simulink model "matlab_physics_demo_model"  (R2022b)
settings: Solver=ode4  StartTime=0.0  StopTime=inf  FixedStep=0.003  RelTol=1e-3
values from neighbouring files (symbols this model uses):
  A1 = 0    [load_quadrotor_simulink_combined_model.m]    (also in load_quadrotor_simulink_physics_model.m; load_quadtiltrotor_simulink_physics_model.m = 0.007)
  Apolar = 0    [load_quadrotor_simulink_combined_model.m]    (also in load_quadrotor_simulink_physics_model.m; load_quadtiltrotor_simulink_physics_model.m = 0.057)
  CD0 = 0    [load_quadrotor_simulink_combined_model.m]    (also in load_quadrotor_simulink_physics_model.m; load_quadtiltrotor_simulink_physics_model.m = 0.022)
  chord = 1    [load_quadrotor_simulink_combined_model.m]    (also in load_quadrotor_simulink_physics_model.m; load_quadtiltrotor_simulink_physics_model.m = 0.351342)
  CL0 = 0    [load_quadrotor_simulink_combined_model.m]    (also in load_quadrotor_simulink_physics_model.m; load_quadtiltrotor_simulink_physics_model.m = 0.38)
  CLa = 0    [load_quadrotor_simulink_combined_model.m]    (also in load_quadrotor_simulink_physics_model.m; load_quadtiltrotor_simulink_physics_model.m = 18.5)
  CLa_dot = 0    [load_quadrotor_simulink_combined_model.m]    (also in load_quadrotor_simulink_physics_model.m; load_quadtiltrotor_simulink_physics_model.m = 2.64)
  Clb = 0    [load_quadrotor_simulink_combined_model.m]    (also in load_quadrotor_simulink_physics_model.m; load_quadtiltrotor_simulink_physics_model.m)
  ClDa = 0    [load_quadrotor_simulink_combined_model.m]    (also in load_quadrotor_simulink_physics_model.m; load_quadtiltrotor_simulink_physics_model.m = 0.1695)
  CLDe = 0    [load_quadrotor_simulink_combined_model.m]    (also in load_quadrotor_simulink_physics_model.m; load_quadtiltrotor_simulink_physics_model.m)
  CLDf = 0    [load_quadrotor_simulink_combined_model.m]    (also in load_quadrotor_simulink_physics_model.m; load_quadtiltrotor_simulink_physics_model.m = 0.4)
  ClDr = 0    [load_quadrotor_simulink_combined_model.m]    (also in load_quadrotor_simulink_physics_model.m; load_quadtiltrotor_simulink_physics_model.m)
  Clp = 0    [load_quadrotor_simulink_combined_model.m]    (also in load_quadrotor_simulink_physics_model.m; load_quadtiltrotor_simulink_physics_model.m)
  CLq = 0    [load_quadrotor_simulink_combined_model.m]    (also in load_quadrotor_simulink_physics_model.m; load_quadtiltrotor_simulink_physics_model.m = 7.4)
  Clr = 0    [load_quadrotor_simulink_combined_model.m]    (also in load_quadrotor_simulink_physics_model.m; load_quadtiltrotor_simulink_physics_model.m)
  Cm0 = 0    [load_quadrotor_simulink_combined_model.m]    (also in load_quadrotor_simulink_physics_model.m; load_quadtiltrotor_simulink_physics_model.m)
  Cma = 0    [load_quadrotor_simulink_combined_model.m]    (also in load_quadrotor_simulink_physics_model.m; load_quadtiltrotor_simulink_physics_model.m)
  CmDe = 0    [load_quadrotor_simulink_combined_model.m]    (also in load_quadrotor_simulink_physics_model.m; load_quadtiltrotor_simulink_physics_model.m = -3.2)
  CmDf = 0    [load_quadrotor_simulink_combined_model.m]    (also in load_quadrotor_simulink_physics_model.m; load_quadtiltrotor_simulink_physics_model.m)
  Cmq = 0    [load_quadrotor_simulink_combined_model.m]    (also in load_quadrotor_simulink_physics_model.m; load_quadtiltrotor_simulink_physics_model.m)
  Cnb = 0    [load_quadrotor_simulink_combined_model.m]    (also in load_quadrotor_simulink_physics_model.m; load_quadtiltrotor_simulink_physics_model.m)
  CnDa = 0    [load_quadrotor_simulink_combined_model.m]    (also in load_quadrotor_simulink_physics_model.m; load_quadtiltrotor_simulink_physics_model.m = -0.023)
  CnDr = 0    [load_quadrotor_simulink_combined_model.m]    (also in load_quadrotor_simulink_physics_model.m; load_quadtiltrotor_simulink_physics_model.m)
  Cnp = 0    [load_quadrotor_simulink_combined_model.m]    (also in load_quadrotor_simulink_physics_model.m; load_quadtiltrotor_simulink_physics_model.m = -0.0889)
  Cnr = 0    [load_quadrotor_simulink_combined_model.m]    (also in load_quadrotor_simulink_physics_model.m; load_quadtiltrotor_simulink_physics_model.m = -0.19997)
  cross_section_area = 1    [load_quadrotor_simulink_combined_model.m]    (also in load_quadrotor_simulink_physics_model.m; load_quadtiltrotor_simulink_physics_model.m = 9.5)
  CYb = 0    [load_quadrotor_simulink_combined_model.m]    (also in load_quadrotor_simulink_physics_model.m; load_quadtiltrotor_simulink_physics_model.m = -1.098)
  CYDr = 0    [load_quadrotor_simulink_combined_model.m]    (also in load_quadrotor_simulink_physics_model.m; load_quadtiltrotor_simulink_physics_model.m = 0.143)
  drag_coeff_angular = -0.5    [load_quadrotor_simulink_combined_model.m]    (also in load_quadrotor_simulink_physics_model.m; load_quadtiltrotor_simulink_physics_model.m = 0.2)
  drag_coeff_linear = -0.5    [load_quadrotor_simulink_combined_model.m]    (also in load_quadrotor_simulink_physics_model.m; load_quadtiltrotor_simulink_physics_model.m = 0.2)
  elarm = 0    [load_quadrotor_simulink_combined_model.m]    (also in load_quadrotor_simulink_physics_model.m; load_quadtiltrotor_simulink_physics_model.m = 0.121)
  enable_FW_forces = 0    [load_quadrotor_simulink_combined_model.m]    (also in load_quadrotor_simulink_physics_model.m; load_quadtiltrotor_simulink_physics_model.m = 1)
  initial_rpy = [0, 0, 0]    [load_quadrotor_simulink_combined_model.m]    (also in load_quadrotor_simulink_physics_model.m; load_quadtiltrotor_simulink_physics_model.m)
  initial_xyz = [0, 0, -4]    [load_quadrotor_simulink_combined_model.m]    (also in load_quadrotor_simulink_physics_model.m; load_quadtiltrotor_simulink_physics_model.m = [2, 3, -4])
  mass = 1    [load_quadrotor_simulink_combined_model.m]    (also in load_quadrotor_simulink_physics_model.m; load_quadtiltrotor_simulink_physics_model.m = 10)
  span = 0    [load_quadrotor_simulink_combined_model.m]    (also in load_quadrotor_simulink_physics_model.m; load_quadtiltrotor_simulink_physics_model.m = 2.795)
libraries: aerolibutil x6, vrlib x4, simulink x3, sharedtransform x2, aerolibasang x2, shared6dof x1, matrix_library x1
(part 2 of 2)

== system matlab_physics_demo_model/Subsystem4/Subsystem3 ==
  wrench : Inport  PortDimensions=9
  Demux{,1..3} (4 alike) : Demux  Outputs=3
  force:x : Outport
  force:y : Outport  Port=2
  force:z : Outport  Port=3
  torque:x : Outport  Port=4
  torque:y : Outport  Port=5
  torque:z : Outport  Port=6
  position:x : Outport  Port=7
  position:y : Outport  Port=8
  position:z : Outport  Port=9
  wires:
  wrench/1 -> Demux2/1
  Demux2/2 -> Demux1/1  "torque"
  Demux1/3 -> torque:z/1
  Demux2/1 -> Demux/1  "force"
  Demux1/1 -> torque:x/1
  Demux/3 -> force:z/1
  Demux/2 -> force:y/1
  Demux1/2 -> torque:y/1
  Demux/1 -> force:x/1
  Demux3/2 -> position:y/1
  Demux3/3 -> position:z/1
  Demux3/1 -> position:x/1
  Demux2/3 -> Demux3/1  "position"

== system matlab_physics_demo_model/Subsystem4/Subsystem4 ==
  wrench : Inport  PortDimensions=9
  Demux{,1..3} (4 alike) : Demux  Outputs=3
  force:x : Outport
  force:y : Outport  Port=2
  force:z : Outport  Port=3
  torque:x : Outport  Port=4
  torque:y : Outport  Port=5
  torque:z : Outport  Port=6
  position:x : Outport  Port=7
  position:y : Outport  Port=8
  position:z : Outport  Port=9
  wires:
  wrench/1 -> Demux2/1
  Demux2/2 -> Demux1/1  "torque"
  Demux1/3 -> torque:z/1
  Demux2/1 -> Demux/1  "force"
  Demux1/1 -> torque:x/1
  Demux/3 -> force:z/1
  Demux/2 -> force:y/1
  Demux1/2 -> torque:y/1
  Demux/1 -> force:x/1
  Demux3/2 -> position:y/1
  Demux3/3 -> position:z/1
  Demux3/1 -> position:x/1
  Demux2/3 -> Demux3/1  "position"

== system matlab_physics_demo_model/Subsystem4/Subsystem5 ==
  wrench : Inport  PortDimensions=9
  Demux{,1..3} (4 alike) : Demux  Outputs=3
  force:x : Outport
  force:y : Outport  Port=2
  force:z : Outport  Port=3
  torque:x : Outport  Port=4
  torque:y : Outport  Port=5
  torque:z : Outport  Port=6
  position:x : Outport  Port=7
  position:y : Outport  Port=8
  position:z : Outport  Port=9
  wires:
  wrench/1 -> Demux2/1
  Demux2/2 -> Demux1/1  "torque"
  Demux1/3 -> torque:z/1
  Demux2/1 -> Demux/1  "force"
  Demux1/1 -> torque:x/1
  Demux/3 -> force:z/1
  Demux/2 -> force:y/1
  Demux1/2 -> torque:y/1
  Demux/1 -> force:x/1
  Demux3/2 -> position:y/1
  Demux3/3 -> position:z/1
  Demux3/1 -> position:x/1
  Demux2/3 -> Demux3/1  "position"

== system matlab_physics_demo_model/Subsystem4/Subsystem6 ==
  wrench : Inport  PortDimensions=9
  Demux{,1..3} (4 alike) : Demux  Outputs=3
  force:x : Outport
  force:y : Outport  Port=2
  force:z : Outport  Port=3
  torque:x : Outport  Port=4
  torque:y : Outport  Port=5
  torque:z : Outport  Port=6
  position:x : Outport  Port=7
  position:y : Outport  Port=8
  position:z : Outport  Port=9
  wires:
  wrench/1 -> Demux2/1
  Demux2/2 -> Demux1/1  "torque"
  Demux1/3 -> torque:z/1
  Demux2/1 -> Demux/1  "force"
  Demux1/1 -> torque:x/1
  Demux/3 -> force:z/1
  Demux/2 -> force:y/1
  Demux1/2 -> torque:y/1
  Demux/1 -> force:x/1
  Demux3/2 -> position:y/1
  Demux3/3 -> position:z/1
  Demux3/1 -> position:x/1
  Demux2/3 -> Demux3/1  "position"

== system matlab_physics_demo_model/Subsystem4/Subsystem7 ==
  wrench : Inport  PortDimensions=9
  Demux{,1..3} (4 alike) : Demux  Outputs=3
  force:x : Outport
  force:y : Outport  Port=2
  force:z : Outport  Port=3
  torque:x : Outport  Port=4
  torque:y : Outport  Port=5
  torque:z : Outport  Port=6
  position:x : Outport  Port=7
  position:y : Outport  Port=8
  position:z : Outport  Port=9
  wires:
  Demux2/3 -> Demux3/1  "position"
  Demux3/1 -> position:x/1
  Demux3/3 -> position:z/1
  Demux3/2 -> position:y/1
  Demux/1 -> force:x/1
  Demux1/2 -> torque:y/1
  Demux/2 -> force:y/1
  Demux/3 -> force:z/1
  Demux1/1 -> torque:x/1
  Demux2/1 -> Demux/1  "force"
  Demux1/3 -> torque:z/1
  Demux2/2 -> Demux1/1  "torque"
  wrench/1 -> Demux2/1

== system matlab_physics_demo_model/Subsystem4/Subsystem8 ==
  wrench : Inport  PortDimensions=9
  Demux{,1..3} (4 alike) : Demux  Outputs=3
  force:x : Outport
  force:y : Outport  Port=2
  force:z : Outport  Port=3
  torque:x : Outport  Port=4
  torque:y : Outport  Port=5
  torque:z : Outport  Port=6
  position:x : Outport  Port=7
  position:y : Outport  Port=8
  position:z : Outport  Port=9
  wires:
  Demux2/3 -> Demux3/1  "position"
  Demux3/1 -> position:x/1
  Demux3/3 -> position:z/1
  Demux3/2 -> position:y/1
  Demux/1 -> force:x/1
  Demux1/2 -> torque:y/1
  Demux/2 -> force:y/1
  Demux/3 -> force:z/1
  Demux1/1 -> torque:x/1
  Demux2/1 -> Demux/1  "force"
  Demux1/3 -> torque:z/1
  Demux2/2 -> Demux1/1  "torque"
  wrench/1 -> Demux2/1

== system matlab_physics_demo_model/Drone Physics Model/AggregateRotorWrenches/Subsystem1 ==
  external_wrench : Inport
  Add10 : Sum
  Add8 : Sum
  Add9 : Sum
  Bus Selector7 : BusSelector  OutputSignals=force:x,force:y,force:z
  Bus Selector8 : BusSelector  OutputSignals=position:x,position:y,position:z
  Bus Selector9 : BusSelector  OutputSignals=torque:x,torque:y,torque:z
  Cross Product : vrlib/Utilities/Cross Product
  Demux : Demux  Outputs=3
  Mux3 : Mux  Inputs=3
  Mux4 : Mux  Inputs=3
  total_torque_x : Outport
  total_torque_y : Outport  Port=2
  total_torque_z : Outport  Port=3
  wires:
  Mux4/1 -> Cross Product/1  "pos"
  Demux/3 -> Add10/2  "torque_from_force_z"
  Demux/2 -> Add9/2  "torque_from_force_y"
  Bus Selector9/2 -> Add9/1  "<torque:y>"
  Bus Selector8/1 -> Mux4/1  "<position:x>"
  Bus Selector7/3 -> Mux3/3  "<force:z>"
  Bus Selector9/1 -> Add8/1  "<torque:x>"
  Mux3/1 -> Cross Product/2  "force"
  Bus Selector7/1 -> Mux3/1  "<force:x>"
  Bus Selector9/3 -> Add10/1  "<torque:z>"
  Cross Product/1 -> Demux/1
  Bus Selector8/3 -> Mux4/3  "<position:z>"
  Bus Selector7/2 -> Mux3/2  "<force:y>"
  Bus Selector8/2 -> Mux4/2  "<position:y>"
  Demux/1 -> Add8/2  "torque_from_force_x"
  Add8/1 -> total_torque_x/1  "total_torque_x"
  Add9/1 -> total_torque_y/1  "total_torque_y"
  external_wrench/1 -> Bus Selector8/1, Bus Selector7/1, Bus Selector9/1
  Add10/1 -> total_torque_z/1  "total_torque_z"

== system matlab_physics_demo_model/Drone Physics Model/AggregateRotorWrenches/Subsystem2 ==
  external_wrench : Inport
  Add10 : Sum
  Add8 : Sum
  Add9 : Sum
  Bus Selector7 : BusSelector  OutputSignals=force:x,force:y,force:z
  Bus Selector8 : BusSelector  OutputSignals=position:x,position:y,position:z
  Bus Selector9 : BusSelector  OutputSignals=torque:x,torque:y,torque:z
  Cross Product : vrlib/Utilities/Cross Product
  Demux : Demux  Outputs=3
  Mux3 : Mux  Inputs=3
  Mux4 : Mux  Inputs=3
  total_torque_x : Outport
  total_torque_y : Outport  Port=2
  total_torque_z : Outport  Port=3
  wires:
  Mux4/1 -> Cross Product/1  "pos"
  Demux/3 -> Add10/2  "torque_from_force_z"
  Demux/2 -> Add9/2  "torque_from_force_y"
  Bus Selector9/2 -> Add9/1  "<torque:y>"
  Bus Selector8/1 -> Mux4/1  "<position:x>"
  Bus Selector7/3 -> Mux3/3  "<force:z>"
  Bus Selector9/1 -> Add8/1  "<torque:x>"
  Mux3/1 -> Cross Product/2  "force"
  Bus Selector7/1 -> Mux3/1  "<force:x>"
  Bus Selector9/3 -> Add10/1  "<torque:z>"
  Cross Product/1 -> Demux/1
  Bus Selector8/3 -> Mux4/3  "<position:z>"
  Bus Selector7/2 -> Mux3/2  "<force:y>"
  Bus Selector8/2 -> Mux4/2  "<position:y>"
  Demux/1 -> Add8/2  "torque_from_force_x"
  Add8/1 -> total_torque_x/1  "total_torque_x"
  Add9/1 -> total_torque_y/1  "total_torque_y"
  external_wrench/1 -> Bus Selector8/1, Bus Selector7/1, Bus Selector9/1
  Add10/1 -> total_torque_z/1  "total_torque_z"

== system matlab_physics_demo_model/Drone Physics Model/AggregateRotorWrenches/Subsystem3 ==
  external_wrench : Inport
  Add10 : Sum
  Add8 : Sum
  Add9 : Sum
  Bus Selector7 : BusSelector  OutputSignals=force:x,force:y,force:z
  Bus Selector8 : BusSelector  OutputSignals=position:x,position:y,position:z
  Bus Selector9 : BusSelector  OutputSignals=torque:x,torque:y,torque:z
  Cross Product : vrlib/Utilities/Cross Product
  Demux : Demux  Outputs=3
  Mux3 : Mux  Inputs=3
  Mux4 : Mux  Inputs=3
  total_torque_x : Outport
  total_torque_y : Outport  Port=2
  total_torque_z : Outport  Port=3
  wires:
  Mux4/1 -> Cross Product/1  "pos"
  Demux/3 -> Add10/2  "torque_from_force_z"
  Demux/2 -> Add9/2  "torque_from_force_y"
  Bus Selector9/2 -> Add9/1  "<torque:y>"
  Bus Selector8/1 -> Mux4/1  "<position:x>"
  Bus Selector7/3 -> Mux3/3  "<force:z>"
  Bus Selector9/1 -> Add8/1  "<torque:x>"
  Mux3/1 -> Cross Product/2  "force"
  Bus Selector7/1 -> Mux3/1  "<force:x>"
  Bus Selector9/3 -> Add10/1  "<torque:z>"
  Cross Product/1 -> Demux/1
  Bus Selector8/3 -> Mux4/3  "<position:z>"
  Bus Selector7/2 -> Mux3/2  "<force:y>"
  Bus Selector8/2 -> Mux4/2  "<position:y>"
  Demux/1 -> Add8/2  "torque_from_force_x"
  Add8/1 -> total_torque_x/1  "total_torque_x"
  Add9/1 -> total_torque_y/1  "total_torque_y"
  external_wrench/1 -> Bus Selector8/1, Bus Selector7/1, Bus Selector9/1
  Add10/1 -> total_torque_z/1  "total_torque_z"

== system matlab_physics_demo_model/Drone Physics Model/AggregateRotorWrenches/Subsystem4 ==
  external_wrench : Inport
  Add10 : Sum
  Add8 : Sum
  Add9 : Sum
  Bus Selector7 : BusSelector  OutputSignals=force:x,force:y,force:z
  Bus Selector8 : BusSelector  OutputSignals=position:x,position:y,position:z
  Bus Selector9 : BusSelector  OutputSignals=torque:x,torque:y,torque:z
  Cross Product : vrlib/Utilities/Cross Product
  Demux : Demux  Outputs=3
  Mux3 : Mux  Inputs=3
  Mux4 : Mux  Inputs=3
  total_torque_x : Outport
  total_torque_y : Outport  Port=2
  total_torque_z : Outport  Port=3
  wires:
  Mux4/1 -> Cross Product/1  "pos"
  Demux/3 -> Add10/2  "torque_from_force_z"
  Demux/2 -> Add9/2  "torque_from_force_y"
  Bus Selector9/2 -> Add9/1  "<torque:y>"
  Bus Selector8/1 -> Mux4/1  "<position:x>"
  Bus Selector7/3 -> Mux3/3  "<force:z>"
  Bus Selector9/1 -> Add8/1  "<torque:x>"
  Mux3/1 -> Cross Product/2  "force"
  Bus Selector7/1 -> Mux3/1  "<force:x>"
  Bus Selector9/3 -> Add10/1  "<torque:z>"
  Cross Product/1 -> Demux/1
  Bus Selector8/3 -> Mux4/3  "<position:z>"
  Bus Selector7/2 -> Mux3/2  "<force:y>"
  Bus Selector8/2 -> Mux4/2  "<position:y>"
  Demux/1 -> Add8/2  "torque_from_force_x"
  Add8/1 -> total_torque_x/1  "total_torque_x"
  Add9/1 -> total_torque_y/1  "total_torque_y"
  external_wrench/1 -> Bus Selector8/1, Bus Selector7/1, Bus Selector9/1
  Add10/1 -> total_torque_z/1  "total_torque_z"

== system matlab_physics_demo_model/Drone Physics Model/IsGrounded/RotateBodyToWorld ==
  q : Inport
  vec_body : Inport  Port=2
  Quaternion Inverse : aerolibutil/Quaternion Inverse
  Quaternion Rotation : aerolibutil/Quaternion Rotation
  vec_world : Outport
  wires:
  Quaternion Rotation/1 -> vec_world/1
  Quaternion Inverse/1 -> Quaternion Rotation/1
  q/1 -> Quaternion Inverse/1
  vec_body/1 -> Quaternion Rotation/2

== system matlab_physics_demo_model/Drone Physics Model/WingForces/Compute Air Data ==
  vel_body : Inport  PortDimensions=3
  air_density : Inport  Port=2
  Bus Creator : BusCreator  Inputs=4
  Dynamic Pressure : aerolibasang/Dynamic Pressure
  "Incidence, Sideslip, & Airspeed" : aerolibasang/Incidence, Sideslip, & Airspeed
  ProtectForDivideByZero : Subsystem
  AirData : Outport  VectorParamsAs1DForOutWhenUnconnected=off
  wires:
  Bus Creator/1 -> AirData/1
  "Incidence, Sideslip, & Airspeed"/1 -> Bus Creator/1  "alpha"
  air_density/1 -> Dynamic Pressure/2
  "Incidence, Sideslip, & Airspeed"/3 -> Bus Creator/3  "airspeed"
  Dynamic Pressure/1 -> Bus Creator/4  "q_dyn"
  "Incidence, Sideslip, & Airspeed"/2 -> Bus Creator/2  "beta"
  vel_body/1 -> ProtectForDivideByZero/1(Vin), Dynamic Pressure/1
  ProtectForDivideByZero/1(Vout) -> "Incidence, Sideslip, & Airspeed"/1

== system matlab_physics_demo_model/Drone Physics Model/WingForces/Compute Body Frame Forces and Moments ==
  AirData : Inport
  CtrlSurfaces : Inport  Port=2
  p,q,r : Inport  Port=3
  Bus Selector : BusSelector  OutputSignals=alpha,beta
  Mux : Mux  Inputs=2
  Rotate FM to body frame : Subsystem
  Wind frame F& M : Subsystem
  F_b : Outport  Unit=kg*m/s^2  VectorParamsAs1DForOutWhenUnconnected=off
  M_b : Outport  Port=2  Unit=kg*m/s  VectorParamsAs1DForOutWhenUnconnected=off
  wires:
  Mux/1 -> Rotate FM to body frame/2(alpha_beta)
  Bus Selector/2 -> Mux/2  "<beta>"
  Bus Selector/1 -> Mux/1  "<alpha>"
  Wind frame F& M/1(FM_w) -> Rotate FM to body frame/1(FM_w)  "FM_W"
  p,q,r/1 -> Wind frame F& M/3(p,q,r)
  Rotate FM to body frame/2(M_b) -> M_b/1
  Rotate FM to body frame/1(F_b) -> F_b/1
  CtrlSurfaces/1 -> Wind frame F& M/2(CtrlSurfaces)
  AirData/1 -> Wind frame F& M/1(Airdata), Bus Selector/1

== system matlab_physics_demo_model/Drone Physics Model/WingForces/Compute Air Data/ProtectForDivideByZero ==
  Vin : Inport
  Dot Product : DotProduct  OutDataTypeStr=Inherit: Inherit via internal rule
  InifinitesimalSpeed : Constant  Value=[ 1e-6 1e-6 1e-6]
      settings: AttributesFormatString=%<Value>
  Sqrt : Sqrt
  Switch : Switch  Criteria=u2 > Threshold  SaturateOnIntegerOverflow=off  InputSameDT=off
  Vout : Outport
  wires:
  Sqrt/1 -> Switch/2
  Vin/1 -> Dot Product/1, Dot Product/2, Switch/1
  Switch/1 -> Vout/1
  InifinitesimalSpeed/1 -> Switch/3
  Dot Product/1 -> Sqrt/1

== system matlab_physics_demo_model/Drone Physics Model/WingForces/Compute Body Frame Forces and Moments/Rotate FM to body frame ==
  FM_w : Inport
  alpha_beta : Inport  Port=2
  BodyForces : Scope
  Forces : Selector  InputPortWidth=6  IndexOptions=Index vector (dialog)  Indices=[1 2 3]  OutputSizes=[(-2)]
  ForcesWorld : Scope
  Moments : Selector  InputPortWidth=6  IndexOptions=Index vector (dialog)  Indices=[4 5 6]  OutputSizes=[(-2)]
  Rotate Forces : Subsystem
  Rotate Moments : Subsystem
  F_b : Outport  VectorParamsAs1DForOutWhenUnconnected=off
  M_b : Outport  Port=2  VectorParamsAs1DForOutWhenUnconnected=off
  wires:
  alpha_beta/1 -> Rotate Forces/2(alpha_beta), Rotate Moments/1(alpha_beta)
  Moments/1 -> Rotate Moments/2(M_w)
  FM_w/1 -> Moments/1, Forces/1
  Forces/1 -> ForcesWorld/1, Rotate Forces/1(F_w)
  Rotate Moments/1(M_b) -> M_b/1
  Rotate Forces/1(F_b) -> BodyForces/1, F_b/1

== system matlab_physics_demo_model/Drone Physics Model/WingForces/Compute Body Frame Forces and Moments/Wind frame F& M ==
  Airdata : Inport
  CtrlSurfaces : Inport  Port=2
  p,q,r : Inport  Port=3
  Bus Creator1 : BusCreator  Inputs=2
  Bus Selector1 : BusSelector  OutputSignals=aileron_angle,rudder_angle
  Bus Selector2 : BusSelector  OutputSignals=elevator_angle,flap_angle
  Bus Selector6 : BusSelector  OutputSignals=beta,airspeed
  Bus Selector7 : BusSelector  OutputSignals=alpha,airspeed
  Get Forces and Moments : Subsystem
  Lateral Channel : Subsystem
  Longitudinal Channel : Subsystem
  FM_w : Outport  PortDimensions=6  VectorParamsAs1DForOutWhenUnconnected=off
  wires:
  Get Forces and Moments/1(FM_w) -> FM_w/1
  Bus Creator1/1 -> Get Forces and Moments/2(AeroCoeffs)
  Bus Selector7/2 -> Longitudinal Channel/2(Airspeed)  "<airspeed>"
  Bus Selector7/1 -> Longitudinal Channel/1(alpha)  "<alpha>"
  Bus Selector6/2 -> Lateral Channel/2(Airspeed)  "<airspeed>"
  Bus Selector6/1 -> Lateral Channel/1(beta)  "<beta>"
  Airdata/1 -> Bus Selector6/1, Bus Selector7/1, Get Forces and Moments/1(Airdata)
  Bus Selector2/2 -> Longitudinal Channel/4(dF)  "<flap_angle>"
  Bus Selector2/1 -> Longitudinal Channel/3(dE)  "<elevator_angle>"
  Bus Selector1/2 -> Lateral Channel/4(dR)  "<rudder_angle>"
  Bus Selector1/1 -> Lateral Channel/3(dA)  "<aileron_angle>"
  CtrlSurfaces/1 -> Bus Selector1/1, Bus Selector2/1
  p,q,r/1 -> Lateral Channel/5(p,q,r), Longitudinal Channel/5(p,q,r)
  Lateral Channel/1(Lateral) -> Bus Creator1/1
  Longitudinal Channel/1(Longitudinal) -> Bus Creator1/2

== system matlab_physics_demo_model/Drone Physics Model/WingForces/Compute Body Frame Forces and Moments/Rotate FM to body frame/Rotate Forces ==
  F_w : Inport
  alpha_beta : Inport  Port=2
  Product2 : Product  Multiplication=Matrix(*)  SaturateOnIntegerOverflow=on  OutDataTypeStr=Inherit: Same as first input
  RB2W : Subsystem
  RW2B : Math  Operator=transpose  SignedPower=on
  F_b : Outport  PortDimensions=3  VectorParamsAs1DForOutWhenUnconnected=off
  wires:
  RW2B/1 -> Product2/1
  F_w/1 -> Product2/2
  Product2/1 -> F_b/1
  alpha_beta/1 -> RB2W/1(aoa beta)
  RB2W/1(Rw2b) -> RW2B/1

== system matlab_physics_demo_model/Drone Physics Model/WingForces/Compute Body Frame Forces and Moments/Rotate FM to body frame/Rotate Moments ==
  alpha_beta : Inport
  M_w : Inport  Port=2
  Product2 : Product  Multiplication=Matrix(*)  SaturateOnIntegerOverflow=on  OutDataTypeStr=Inherit: Same as first input
  RB2W : Subsystem
  RW2B : Math  Operator=transpose  SignedPower=on
  M_b : Outport  PortDimensions=3  VectorParamsAs1DForOutWhenUnconnected=off
  wires:
  RW2B/1 -> Product2/1
  RB2W/1(Rw2b) -> RW2B/1
  alpha_beta/1 -> RB2W/1(aoa beta)
  Product2/1 -> M_b/1
  M_w/1 -> Product2/2

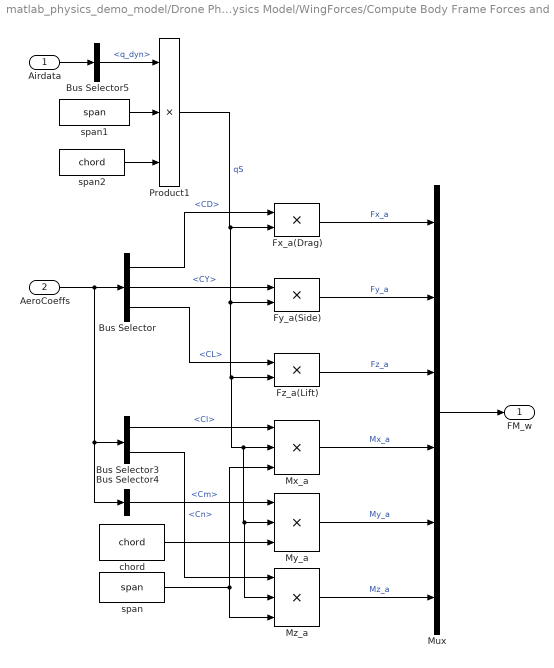
== system matlab_physics_demo_model/Drone Physics Model/WingForces/Compute Body Frame Forces and Moments/Wind frame F& M/Get Forces and Moments ==
  Airdata : Inport
  AeroCoeffs : Inport  Port=2
  Bus Selector : BusSelector  OutputSignals=signal2.CD,signal1.CY,signal2.CL
  Bus Selector3 : BusSelector  OutputSignals=signal1.Cl,signal1.Cn
  Bus Selector4 : BusSelector  OutputSignals=signal2.Cm
  Bus Selector5 : BusSelector  OutputSignals=q_dyn
  Fx_a(Drag) : Product  Inputs=**  SaturateOnIntegerOverflow=on  OutDataTypeStr=Inherit: Same as first input
  Fy_a(Side) : Product  SaturateOnIntegerOverflow=on  OutDataTypeStr=Inherit: Same as first input
  Fz_a(Lift) : Product  SaturateOnIntegerOverflow=on  OutDataTypeStr=Inherit: Same as first input
  Mux : Mux  Inputs=6
  Mx_a : Product  Inputs=3  SaturateOnIntegerOverflow=on  OutDataTypeStr=Inherit: Same as first input
  My_a : Product  Inputs=3  SaturateOnIntegerOverflow=on  OutDataTypeStr=Inherit: Same as first input
  Mz_a : Product  Inputs=3  SaturateOnIntegerOverflow=on  OutDataTypeStr=Inherit: Same as first input
  Product1 : Product  Inputs=3  SaturateOnIntegerOverflow=on  OutDataTypeStr=Inherit: Same as first input
  chord : Constant  Value=chord  VectorParams1D=off
      settings: AttributesFormatString=%<Value>
  span : Constant  Value=span  VectorParams1D=off
      settings: AttributesFormatString=%<Value>
  span1 : Constant  Value=span  VectorParams1D=off
      settings: AttributesFormatString=%<Value>
  span2 : Constant  Value=chord  VectorParams1D=off
      settings: AttributesFormatString=%<Value>
  FM_w : Outport  VectorParamsAs1DForOutWhenUnconnected=off
  wires:
  Mx_a/1 -> Mux/4  "Mx_a"
  Bus Selector/2 -> Fy_a(Side)/1  "<CY>"
  Bus Selector4/1 -> My_a/1  "<Cm>"
  span2/1 -> Product1/3
  Fx_a(Drag)/1 -> Mux/1  "Fx_a"
  Bus Selector/1 -> Fx_a(Drag)/1  "<CD>"
  AeroCoeffs/1 -> Bus Selector/1, Bus Selector4/1, Bus Selector3/1
  My_a/1 -> Mux/5  "My_a"
  Fz_a(Lift)/1 -> Mux/3  "Fz_a"
  Mz_a/1 -> Mux/6  "Mz_a"
  Airdata/1 -> Bus Selector5/1
  chord/1 -> My_a/3
  span/1 -> Mz_a/3, Mx_a/3
  Fy_a(Side)/1 -> Mux/2  "Fy_a"
  Mux/1 -> FM_w/1
  Bus Selector3/2 -> Mz_a/1  "<Cn>"
  Bus Selector/3 -> Fz_a(Lift)/1  "<CL>"
  Product1/1 -> Fx_a(Drag)/2, Fy_a(Side)/2, Fz_a(Lift)/2, Mx_a/2, My_a/2, Mz_a/2  "qS"
  span1/1 -> Product1/2
  Bus Selector3/1 -> Mx_a/1  "<Cl>"
  Bus Selector5/1 -> Product1/1  "<q_dyn>"

== system matlab_physics_demo_model/Drone Physics Model/WingForces/Compute Body Frame Forces and Moments/Wind frame F& M/Lateral Channel ==
  beta : Inport
  Airspeed : Inport  Port=2
  dA : Inport  Port=3
  dR : Inport  Port=4
  p,q,r : Inport  Port=5
  Bus Creator : BusCreator  Inputs=3
  CY : Subsystem
  Cl : Subsystem
  Cn : Subsystem
  Lateral : Outport  VectorParamsAs1DForOutWhenUnconnected=off
  wires:
  Cl/1(Cl) -> Bus Creator/2  "Cl"
  p,q,r/1 -> Cn/4(p,q,r), Cl/4(p,q,r)
  Airspeed/1 -> Cn/5(Airspeed), Cl/5(Airspeed)
  dR/1 -> CY/2(dR), Cl/3(dR), Cn/3(Dr)
  dA/1 -> Cl/2(dA), Cn/2(dA)
  beta/1 -> CY/1(beta), Cl/1(beta), Cn/1(beta)
  Cn/1(Cn) -> Bus Creator/3  "Cn"
  CY/1(CY) -> Bus Creator/1  "CY"
  Bus Creator/1 -> Lateral/1

== system matlab_physics_demo_model/Drone Physics Model/WingForces/Compute Body Frame Forces and Moments/Wind frame F& M/Longitudinal Channel ==
  alpha : Inport
  Airspeed : Inport  Port=2
  dE : Inport  Port=3
  dF : Inport  Port=4
  p,q,r : Inport  Port=5
  Bus Creator : BusCreator  Inputs=3
  CD : Subsystem
  CL : Subsystem
  Cm : Subsystem
  Transfer Fcn : TransferFcn  Numerator=[1 0]  Denominator=[0.1 1]
  Y-down : Gain  Gain=-1  SaturateOnIntegerOverflow=on  OutDataTypeStr=Inherit: Same as input  ParamDataTypeStr=Inherit: Same as input
      settings: AttributesFormatString=%<Gain>
  Longitudinal : Outport  VectorParamsAs1DForOutWhenUnconnected=off
  wires:
  Transfer Fcn/1 -> CL/2(alpha_dot)
  Airspeed/1 -> CL/6(Airspeed)
  p,q,r/1 -> Cm/4(p,q,r), CL/5(p,q,r)
  dF/1 -> Cm/3(Df), CL/4(dF)
  Bus Creator/1 -> Longitudinal/1
  Cm/1(Cm) -> Bus Creator/3  "Cm"
  CL/1(CL) -> CD/1(CL), Y-down/1
  dE/1 -> Cm/2(De), CL/3(dE)
  Y-down/1 -> Bus Creator/2  "CL"
  CD/1(CD) -> Bus Creator/1  "CD"
  alpha/1 -> Transfer Fcn/1, Cm/1(alpha), CL/1(alpha)

== system matlab_physics_demo_model/Drone Physics Model/WingForces/Compute Body Frame Forces and Moments/Rotate FM to body frame/Rotate Forces/RB2W ==
  aoa beta : Inport
  11 : Fcn  Expr=u[3]*u[4]
  12 : Fcn  Expr=u[2]
  13 : Fcn  Expr=u[1]*u[4]
  21 : Fcn  Expr=-u[3]*u[2]
  22 : Fcn  Expr=u[4]
  23 : Fcn  Expr=-u[1]*u[2]
  31 : Fcn  Expr=-u[1]
  32 : Fcn  Expr=0
  33 : Fcn  Expr=u[3]
  Mux : Mux  Inputs=2
  Mux3 : Mux  Inputs=9
  Reshape 9x1->3x3 : Reshape  OutputDimensionality=Customize  OutputDimensions=[3,3]
  sincos : Trigonometry  Operator=sincos
  Rw2b : Outport  VectorParamsAs1DForOutWhenUnconnected=off
  wires:
  Mux/1 -> 11/1, 21/1, 31/1, 12/1, 22/1, 32/1, 13/1, 23/1, 33/1
  aoa beta/1 -> sincos/1
  sincos/2 -> Mux/2
  sincos/1 -> Mux/1
  33/1 -> Mux3/9
  23/1 -> Mux3/8
  13/1 -> Mux3/7
  32/1 -> Mux3/6
  22/1 -> Mux3/5
  12/1 -> Mux3/4
  31/1 -> Mux3/3
  21/1 -> Mux3/2
  11/1 -> Mux3/1
  Reshape 9x1->3x3/1 -> Rw2b/1
  Mux3/1 -> Reshape 9x1->3x3/1

== system matlab_physics_demo_model/Drone Physics Model/WingForces/Compute Body Frame Forces and Moments/Rotate FM to body frame/Rotate Moments/RB2W ==
  aoa beta : Inport
  11 : Fcn  Expr=u[3]*u[4]
  12 : Fcn  Expr=u[2]
  13 : Fcn  Expr=u[1]*u[4]
  21 : Fcn  Expr=-u[3]*u[2]
  22 : Fcn  Expr=u[4]
  23 : Fcn  Expr=-u[1]*u[2]
  31 : Fcn  Expr=-u[1]
  32 : Fcn  Expr=0
  33 : Fcn  Expr=u[3]
  Mux : Mux  Inputs=2
  Mux3 : Mux  Inputs=9
  Reshape 9x1->3x3 : Reshape  OutputDimensionality=Customize  OutputDimensions=[3,3]
  sincos : Trigonometry  Operator=sincos
  Rw2b : Outport  VectorParamsAs1DForOutWhenUnconnected=off
  wires:
  Mux/1 -> 11/1, 21/1, 31/1, 12/1, 22/1, 32/1, 13/1, 23/1, 33/1
  aoa beta/1 -> sincos/1
  sincos/2 -> Mux/2
  sincos/1 -> Mux/1
  33/1 -> Mux3/9
  23/1 -> Mux3/8
  13/1 -> Mux3/7
  32/1 -> Mux3/6
  22/1 -> Mux3/5
  12/1 -> Mux3/4
  31/1 -> Mux3/3
  21/1 -> Mux3/2
  11/1 -> Mux3/1
  Reshape 9x1->3x3/1 -> Rw2b/1
  Mux3/1 -> Reshape 9x1->3x3/1

== system matlab_physics_demo_model/Drone Physics Model/WingForces/Compute Body Frame Forces and Moments/Wind frame F& M/Lateral Channel/CY ==
  beta : Inport
  dR : Inport  Port=2
  CYDr : Constant  Value=CYDr
      settings: AttributesFormatString=%<Value>
  CYb : Constant  Value=CYb
      settings: AttributesFormatString=%<Value>
  Product : Product  SaturateOnIntegerOverflow=on  OutDataTypeStr=Inherit: Same as first input
  Product1 : Product  SaturateOnIntegerOverflow=on  OutDataTypeStr=Inherit: Same as first input
  Sum2 : Sum  SaturateOnIntegerOverflow=on
  CY : Outport  VectorParamsAs1DForOutWhenUnconnected=off
  wires:
  Product1/1 -> Sum2/2
  dR/1 -> Product1/2
  CYDr/1 -> Product1/1
  Product/1 -> Sum2/1
  Sum2/1 -> CY/1
  beta/1 -> Product/2
  CYb/1 -> Product/1

== system matlab_physics_demo_model/Drone Physics Model/WingForces/Compute Body Frame Forces and Moments/Wind frame F& M/Lateral Channel/Cl ==
  beta : Inport
  dA : Inport  Port=2
  dR : Inport  Port=3
  p,q,r : Inport  Port=4
  Airspeed : Inport  Port=5
  ClDa : Constant  Value=ClDa
      settings: AttributesFormatString=%<Value>
  ClDr : Constant  Value=ClDr
      settings: AttributesFormatString=%<Value>
  Clb : Constant  Value=Clb
      settings: AttributesFormatString=%<Value>
  Product1 : Product  SaturateOnIntegerOverflow=on  OutDataTypeStr=Inherit: Same as first input
  Product4 : Product  SaturateOnIntegerOverflow=on  OutDataTypeStr=Inherit: Same as first input
  Product5 : Product  SaturateOnIntegerOverflow=on  OutDataTypeStr=Inherit: Same as first input
  Sum : Sum  Inputs=+++++  SaturateOnIntegerOverflow=on
  roll factors : Subsystem
  Cl : Outport  VectorParamsAs1DForOutWhenUnconnected=off
  wires:
  roll factors/1(Clp) -> Sum/4
  Product5/1 -> Sum/2  "CldA"
  Airspeed/1 -> roll factors/2(Airspeed)
  p,q,r/1 -> roll factors/1(p,q,r)
  roll factors/2(Clr) -> Sum/5
  Product1/1 -> Sum/3  "Cldr"
  Product4/1 -> Sum/1  "Clb"
  Sum/1 -> Cl/1
  dR/1 -> Product1/2
  ClDr/1 -> Product1/1
  dA/1 -> Product5/2
  ClDa/1 -> Product5/1
  beta/1 -> Product4/2
  Clb/1 -> Product4/1

== system matlab_physics_demo_model/Drone Physics Model/WingForces/Compute Body Frame Forces and Moments/Wind frame F& M/Lateral Channel/Cn ==
  note: Cnb too large, creates unfavorable yaw torque in MR mode
  beta : Inport
  dA : Inport  Port=2
  Dr : Inport  Port=3
  p,q,r : Inport  Port=4
  Airspeed : Inport  Port=5
  CnDa : Constant  Value=CnDa
      settings: AttributesFormatString=%<Value>
  CnDr : Constant  Value=CnDr
      settings: AttributesFormatString=%<Value>
  Cnb : Constant  Value=Cnb
      settings: AttributesFormatString=%<Value>
  Product1 : Product  SaturateOnIntegerOverflow=on  OutDataTypeStr=Inherit: Same as first input
  Product4 : Product  SaturateOnIntegerOverflow=on  OutDataTypeStr=Inherit: Same as first input
  Product5 : Product  SaturateOnIntegerOverflow=on  OutDataTypeStr=Inherit: Same as first input
  Sum : Sum  Inputs=+++++  SaturateOnIntegerOverflow=on
  yaw factors : Subsystem
  Cn : Outport  VectorParamsAs1DForOutWhenUnconnected=off
  wires:
  Airspeed/1 -> yaw factors/2(Airspeed)
  p,q,r/1 -> yaw factors/1(p,q,r)
  Cnb/1 -> Product4/1
  beta/1 -> Product4/2
  CnDa/1 -> Product5/1
  Product5/1 -> Sum/2
  dA/1 -> Product5/2
  CnDr/1 -> Product1/1
  Dr/1 -> Product1/2
  Sum/1 -> Cn/1
  Product1/1 -> Sum/3
  yaw factors/1(Cnp) -> Sum/4
  Product4/1 -> Sum/1
  yaw factors/2(Cnr) -> Sum/5

== system matlab_physics_demo_model/Drone Physics Model/WingForces/Compute Body Frame Forces and Moments/Wind frame F& M/Longitudinal Channel/CD ==
  CL : Inport
  Apolar : Constant  Value=A1
      settings: AttributesFormatString=%<Value>
  Apolar (A2) : Constant  Value=Apolar
      settings: AttributesFormatString=%<Value>
  CD0 : Constant  Value=CD0
      settings: AttributesFormatString=%<Value>
  Gain : Gain  Gain=-1  SaturateOnIntegerOverflow=on  OutDataTypeStr=Inherit: Same as input  ParamDataTypeStr=Inherit: Same as input
      settings: AttributesFormatString=%<Gain>
  Math Function : Math  Operator=square  SignedPower=on
  Product : Product  SaturateOnIntegerOverflow=on  OutDataTypeStr=Inherit: Same as first input
  Product1 : Product  SaturateOnIntegerOverflow=on  OutDataTypeStr=Inherit: Same as first input
  Sum1 : Sum  Inputs=+++  SaturateOnIntegerOverflow=on
  CD : Outport  VectorParamsAs1DForOutWhenUnconnected=off
  wires:
  Gain/1 -> CD/1
  Apolar (A2)/1 -> Product/1
  Math Function/1 -> Product/2
  Product1/1 -> Sum1/3
  Product/1 -> Sum1/2
  CL/1 -> Math Function/1, Product1/1
  Sum1/1 -> Gain/1
  CD0/1 -> Sum1/1
  Apolar/1 -> Product1/2

== system matlab_physics_demo_model/Drone Physics Model/WingForces/Compute Body Frame Forces and Moments/Wind frame F& M/Longitudinal Channel/CL ==
  alpha : Inport
  alpha_dot : Inport  Port=2
  dE : Inport  Port=3
  dF : Inport  Port=4
  p,q,r : Inport  Port=5
  Airspeed : Inport  Port=6
  CL0 : Constant  Value=CL0
      settings: AttributesFormatString=%<Value>
  CLDe : Constant  Value=CLDe
      settings: AttributesFormatString=%<Value>
  CLa : Constant  Value=CLa
      settings: AttributesFormatString=%<Value>
  CLa_dot : Constant  Value=CLa_dot
      settings: AttributesFormatString=%<Value>
  CmDe1 : Constant  Value=CLDf
      settings: AttributesFormatString=%<Value>
  Lift due to pitch rate : Subsystem
  Product{1..2,4..5} (4 alike) : Product  SaturateOnIntegerOverflow=on  OutDataTypeStr=Inherit: Same as first input
  Sum : Sum  Inputs=++++++  SaturateOnIntegerOverflow=on
  CL : Outport  VectorParamsAs1DForOutWhenUnconnected=off
  wires:
  CL0/1 -> Sum/1
  Airspeed/1 -> Lift due to pitch rate/2(Airspeed)
  p,q,r/1 -> Lift due to pitch rate/1(p,q,r)
  Lift due to pitch rate/1(CLq) -> Sum/6
  Product2/1 -> Sum/5
  Product5/1 -> Sum/3
  CmDe1/1 -> Product2/1
  dF/1 -> Product2/2
  Sum/1 -> CL/1
  dE/1 -> Product1/2
  CLDe/1 -> Product1/1
  alpha_dot/1 -> Product5/2
  CLa_dot/1 -> Product5/1
  alpha/1 -> Product4/2
  CLa/1 -> Product4/1
  Product4/1 -> Sum/2
  Product1/1 -> Sum/4

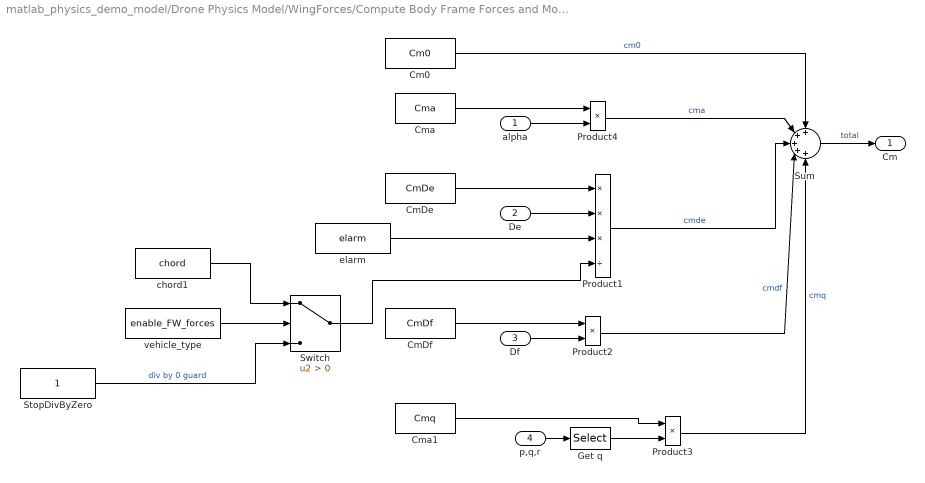
== system matlab_physics_demo_model/Drone Physics Model/WingForces/Compute Body Frame Forces and Moments/Wind frame F& M/Longitudinal Channel/Cm ==
  alpha : Inport
  De : Inport  Port=2
  Df : Inport  Port=3
  p,q,r : Inport  Port=4
  Cm0 : Constant  Value=Cm0
      settings: AttributesFormatString=%<Value>
  CmDe : Constant  Value=CmDe
      settings: AttributesFormatString=%<Value>
  CmDf : Constant  Value=CmDf
      settings: AttributesFormatString=%<Value>
  Cma : Constant  Value=Cma
      settings: AttributesFormatString=%<Value>
  Cma1 : Constant  Value=Cmq
      settings: AttributesFormatString=%<Value>
  Get q : Selector  InputPortWidth=3  IndexOptions=Index vector (dialog)  Indices=2  OutputSizes=[(-2)]
  Product1 : Product  Inputs=***/  SaturateOnIntegerOverflow=on  OutDataTypeStr=Inherit: Same as first input
  Product2 : Product  SaturateOnIntegerOverflow=on  OutDataTypeStr=Inherit: Same as first input
  Product3 : Product  SaturateOnIntegerOverflow=on  OutDataTypeStr=Inherit: Same as first input
  Product4 : Product  SaturateOnIntegerOverflow=on  OutDataTypeStr=Inherit: Same as first input
  StopDivByZero : Constant
      settings: AttributesFormatString=%<Value>
  Sum : Sum  Inputs=+++++  SaturateOnIntegerOverflow=on
  Switch : Switch  Criteria=u2 > Threshold  SaturateOnIntegerOverflow=off  InputSameDT=off
  chord1 : Constant  Value=chord
      settings: AttributesFormatString=%<Value>
  elarm : Constant  Value=elarm
      settings: AttributesFormatString=%<Value>
  vehicle_type : Constant  Value=enable_FW_forces
  Cm : Outport  VectorParamsAs1DForOutWhenUnconnected=off
  wires:
  Switch/1 -> Product1/4
  Get q/1 -> Product3/2
  Product3/1 -> Sum/5  "cmq"
  p,q,r/1 -> Get q/1
  Cma1/1 -> Product3/1
  Product1/1 -> Sum/3  "cmde"
  Product4/1 -> Sum/2  "cma"
  Sum/1 -> Cm/1  "total"
  De/1 -> Product1/2
  CmDe/1 -> Product1/1
  alpha/1 -> Product4/2
  Cma/1 -> Product4/1
  Df/1 -> Product2/2
  CmDf/1 -> Product2/1
  Product2/1 -> Sum/4  "cmdf"
  Cm0/1 -> Sum/1  "cm0"
  elarm/1 -> Product1/3
  vehicle_type/1 -> Switch/2
  StopDivByZero/1 -> Switch/3  "div by 0 guard"
  chord1/1 -> Switch/1

== system matlab_physics_demo_model/Drone Physics Model/WingForces/Compute Body Frame Forces and Moments/Wind frame F& M/Lateral Channel/Cl/roll factors ==
  p,q,r : Inport
  Airspeed : Inport  Port=2
  Constant : Constant  Value=Clp
      settings: AttributesFormatString=%<Value>
  Constant1 : Constant  Value=Clr
      settings: AttributesFormatString=%<Value>
  Get p : Selector  InputPortWidth=3  IndexOptions=Index vector (dialog)  Indices=1  OutputSizes=[(-2)]
  Get r : Selector  InputPortWidth=3  IndexOptions=Index vector (dialog)  Indices=3  OutputSizes=[(-2)]
  Product : Product  SaturateOnIntegerOverflow=on  OutDataTypeStr=Inherit: Same as first input
  Product1 : Product  SaturateOnIntegerOverflow=on  OutDataTypeStr=Inherit: Same as first input
  roll rate fact : Subsystem
  yaw rate fact : Subsystem
  Clp : Outport  VectorParamsAs1DForOutWhenUnconnected=off
  Clr : Outport  Port=2  VectorParamsAs1DForOutWhenUnconnected=off
  wires:
  Get r/1 -> yaw rate fact/1(r)
  p,q,r/1 -> Get r/1, Get p/1
  Get p/1 -> roll rate fact/1(p)
  Airspeed/1 -> yaw rate fact/2(Airspeed), roll rate fact/2(Airspeed)
  yaw rate fact/1(Yaw Rate Fac) -> Product1/2
  Constant1/1 -> Product1/1
  roll rate fact/1(Roll Rate Fac) -> Product/2
  Constant/1 -> Product/1
  Product1/1 -> Clr/1
  Product/1 -> Clp/1

== system matlab_physics_demo_model/Drone Physics Model/WingForces/Compute Body Frame Forces and Moments/Wind frame F& M/Lateral Channel/Cn/yaw factors ==
  p,q,r : Inport
  Airspeed : Inport  Port=2
  Constant : Constant  Value=Cnp
      settings: AttributesFormatString=%<Value>
  Constant1 : Constant  Value=Cnr
      settings: AttributesFormatString=%<Value>
  Get p : Selector  InputPortWidth=3  IndexOptions=Index vector (dialog)  Indices=1  OutputSizes=[(-2)]
  Get r : Selector  InputPortWidth=3  IndexOptions=Index vector (dialog)  Indices=3  OutputSizes=[(-2)]
  Product : Product  SaturateOnIntegerOverflow=on  OutDataTypeStr=Inherit: Same as first input
  Product1 : Product  SaturateOnIntegerOverflow=on  OutDataTypeStr=Inherit: Same as first input
  roll rate fact : Subsystem
  yaw rate fact : Subsystem
  Cnp : Outport  VectorParamsAs1DForOutWhenUnconnected=off
  Cnr : Outport  Port=2  VectorParamsAs1DForOutWhenUnconnected=off
  wires:
  Airspeed/1 -> yaw rate fact/2(Airspeed), roll rate fact/2(Airspeed)
  Get r/1 -> yaw rate fact/1(r)
  p,q,r/1 -> Get r/1, Get p/1
  Get p/1 -> roll rate fact/1(p)
  roll rate fact/1(Roll Rate Fac) -> Product/2
  Constant/1 -> Product/1
  yaw rate fact/1(Yaw Rate Fac) -> Product1/2
  Constant1/1 -> Product1/1
  Product1/1 -> Cnr/1
  Product/1 -> Cnp/1

== system matlab_physics_demo_model/Drone Physics Model/WingForces/Compute Body Frame Forces and Moments/Wind frame F& M/Longitudinal Channel/CL/Lift due to pitch rate ==
  p,q,r : Inport
  Airspeed : Inport  Port=2
  Constant : Constant  Value=CLq
      settings: AttributesFormatString=%<Value>
  Get q : Selector  InputPortWidth=3  IndexOptions=Index vector (dialog)  Indices=2  OutputSizes=[(-2)]
  Product : Product  SaturateOnIntegerOverflow=on  OutDataTypeStr=Inherit: Same as first input
  pitch rate factor : Subsystem
  CLq : Outport  VectorParamsAs1DForOutWhenUnconnected=off
  wires:
  Airspeed/1 -> pitch rate factor/2(Airspeed)
  Get q/1 -> pitch rate factor/1(q)
  p,q,r/1 -> Get q/1
  Product/1 -> CLq/1
  pitch rate factor/1(Pitch Rate Fac) -> Product/2
  Constant/1 -> Product/1

== system matlab_physics_demo_model/Drone Physics Model/WingForces/Compute Body Frame Forces and Moments/Wind frame F& M/Lateral Channel/Cl/roll factors/roll rate fact ==
  p : Inport
  Airspeed : Inport  Port=2
  Cmq1 : Constant  Value=.5
      settings: AttributesFormatString=%<Value>
  Cmq2 : Constant  Value=span
      settings: AttributesFormatString=%<Value>
  Product : Product  Inputs=***/  SaturateOnIntegerOverflow=on  OutDataTypeStr=Inherit: Same as first input
  Saturation : Saturate  UpperLimit=inf  LowerLimit=0.1
      settings: AttributesFormatString="[%<LowerLimit>  %<UpperLimit>]"
  Roll Rate Fac : Outport  VectorParamsAs1DForOutWhenUnconnected=off
  wires:
  Saturation/1 -> Product/4
  Airspeed/1 -> Saturation/1
  Cmq2/1 -> Product/3
  Cmq1/1 -> Product/2
  p/1 -> Product/1
  Product/1 -> Roll Rate Fac/1

== system matlab_physics_demo_model/Drone Physics Model/WingForces/Compute Body Frame Forces and Moments/Wind frame F& M/Lateral Channel/Cl/roll factors/yaw rate fact ==
  r : Inport
  Airspeed : Inport  Port=2
  Cmq1 : Constant  Value=.5
      settings: AttributesFormatString=%<Value>
  Cmq2 : Constant  Value=span
      settings: AttributesFormatString=%<Value>
  Product : Product  Inputs=***/  SaturateOnIntegerOverflow=on  OutDataTypeStr=Inherit: Same as first input
  Saturation : Saturate  UpperLimit=inf  LowerLimit=0.1
      settings: AttributesFormatString="[%<LowerLimit>  %<UpperLimit>]"
  Yaw Rate Fac : Outport  VectorParamsAs1DForOutWhenUnconnected=off
  wires:
  Saturation/1 -> Product/4
  Airspeed/1 -> Saturation/1
  Cmq2/1 -> Product/3
  Cmq1/1 -> Product/2
  r/1 -> Product/1
  Product/1 -> Yaw Rate Fac/1

== system matlab_physics_demo_model/Drone Physics Model/WingForces/Compute Body Frame Forces and Moments/Wind frame F& M/Lateral Channel/Cn/yaw factors/roll rate fact ==
  p : Inport
  Airspeed : Inport  Port=2
  Cmq1 : Constant  Value=.5
      settings: AttributesFormatString=%<Value>
  Cmq2 : Constant  Value=span
      settings: AttributesFormatString=%<Value>
  Product : Product  Inputs=***/  SaturateOnIntegerOverflow=on  OutDataTypeStr=Inherit: Same as first input
  Saturation : Saturate  UpperLimit=inf  LowerLimit=0.1
      settings: AttributesFormatString="[%<LowerLimit>  %<UpperLimit>]"
  Roll Rate Fac : Outport  VectorParamsAs1DForOutWhenUnconnected=off
  wires:
  Saturation/1 -> Product/4
  Airspeed/1 -> Saturation/1
  Cmq2/1 -> Product/3
  Cmq1/1 -> Product/2
  p/1 -> Product/1
  Product/1 -> Roll Rate Fac/1

== system matlab_physics_demo_model/Drone Physics Model/WingForces/Compute Body Frame Forces and Moments/Wind frame F& M/Lateral Channel/Cn/yaw factors/yaw rate fact ==
  r : Inport
  Airspeed : Inport  Port=2
  Cmq1 : Constant  Value=.5
      settings: AttributesFormatString=%<Value>
  Cmq2 : Constant  Value=span
      settings: AttributesFormatString=%<Value>
  Product : Product  Inputs=***/  SaturateOnIntegerOverflow=on  OutDataTypeStr=Inherit: Same as first input
  Saturation : Saturate  UpperLimit=inf  LowerLimit=0.1
      settings: AttributesFormatString="[%<LowerLimit>  %<UpperLimit>]"
  Yaw Rate Fac : Outport  VectorParamsAs1DForOutWhenUnconnected=off
  wires:
  Saturation/1 -> Product/4
  Airspeed/1 -> Saturation/1
  Cmq2/1 -> Product/3
  Cmq1/1 -> Product/2
  r/1 -> Product/1
  Product/1 -> Yaw Rate Fac/1

== system matlab_physics_demo_model/Drone Physics Model/WingForces/Compute Body Frame Forces and Moments/Wind frame F& M/Longitudinal Channel/CL/Lift due to pitch rate/pitch rate factor ==
  q : Inport
  Airspeed : Inport  Port=2
  Cmq2 : Constant  Value=chord
      settings: AttributesFormatString=%<Value>
  Product : Product  Inputs=**/  SaturateOnIntegerOverflow=on  OutDataTypeStr=Inherit: Same as first input
  Saturation : Saturate  UpperLimit=inf  LowerLimit=0.1
      settings: AttributesFormatString="[%<LowerLimit>  %<UpperLimit>]"
  Pitch Rate Fac : Outport  VectorParamsAs1DForOutWhenUnconnected=off
  wires:
  Saturation/1 -> Product/3
  Cmq2/1 -> Product/2
  Airspeed/1 -> Saturation/1
  q/1 -> Product/1
  Product/1 -> Pitch Rate Fac/1
